simulink model "lstm_model_test"  (R2024b)
settings: Solver=VariableStepAuto  StartTime=0.0  StopTime=50  RelTol=1e-3
values from neighbouring files (symbols this model uses):
  C = ft .* C + it .* Ct_candidate    [lstm_first_principle.m]
libraries: deeplib x1
settings Model: Creator=HP  LastModifiedBy=HP
settings DebuggingCC: SigSpecEnsureSampleTimeMsg=none

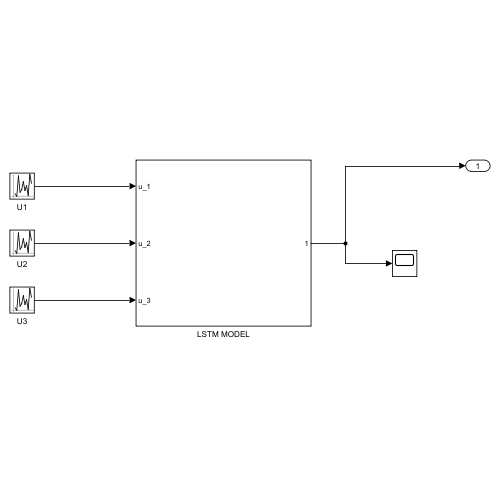
[thumbnail: Simulink's stored preview of the top-level diagram]
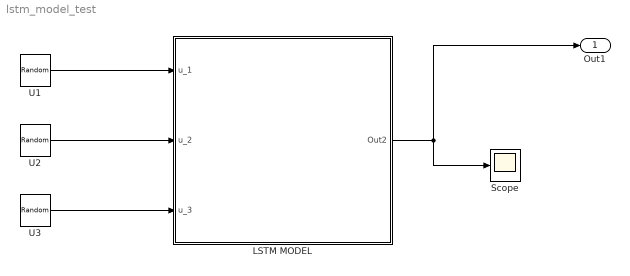
== system lstm_model_test ==
  LSTM MODEL : Subsystem
  Scope : Scope
  U1 : UniformRandomNumber  Minimum=0  Maximum=50  SampleTime=0.1
  U2 : UniformRandomNumber  Minimum=0  Maximum=50  SampleTime=0.1
  U3 : UniformRandomNumber  Minimum=0  Maximum=50  SampleTime=0.1
  Out1 : Outport
  wires:
  U1/1 -> LSTM MODEL/1(u_1)
  U2/1 -> LSTM MODEL/2(u_2)
  U3/1 -> LSTM MODEL/3(u_3)
  LSTM MODEL/1(Out2) -> Out1/1, Scope/1

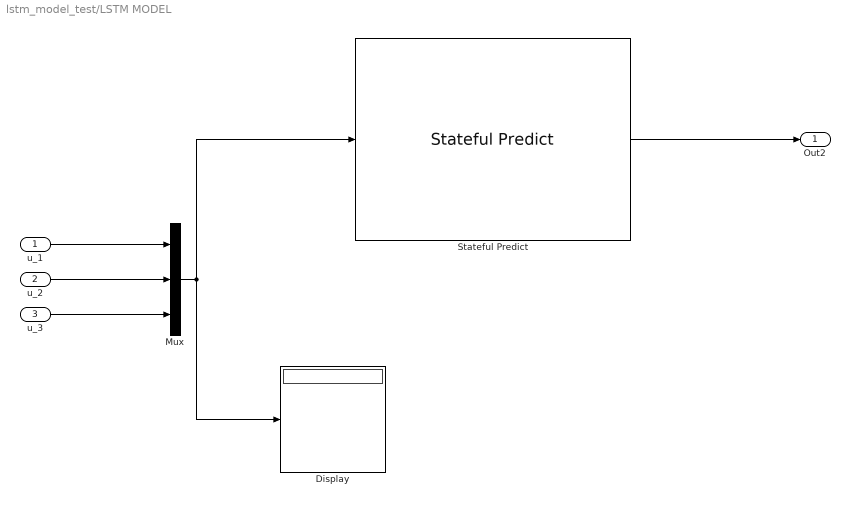
== system lstm_model_test/LSTM MODEL ==
  u_1 : Inport
  u_2 : Inport  Port=2
  u_3 : Inport  Port=3
  Display : Display
  Mux : Mux  Inputs=3
  Stateful Predict : deeplib/Stateful Predict  Network=Network from MAT-file  NetworkFunction=untitled  NetworkFilePath=C:\Users\HP\Desktop\LSTM\lstm_model.mat  InputDataFormats={'',''}  SampleTime=50  ForceInterpretedSim=off  EnableDLNetwork=on  LastKnownNetworkFilePath=''  LastKnownNetworkTimeStamp=''
  Out2 : Outport
  wires:
  u_3/1 -> Mux/3
  Stateful Predict/1 -> Out2/1
  Mux/1 -> Display/1, Stateful Predict/1
  u_1/1 -> Mux/1
  u_2/1 -> Mux/2
